simulink model "Id_u_d"  (Simulink 7.1)
settings: Solver=ode4  StartTime=0.0  StopTime=6.0  FixedStep=0.001  RelTol=1e-3
settings Model: Creator=Orlo  LastModifiedBy=Orlo
settings OptimizationCC: InlineInvariantSignals=on
settings DebuggingCC: SaveWithParameterizedLinksMsg=none  SignalResolutionControl=TryResolveAllWithWarning  MultiTaskDSMMsg=warning  MultiTaskCondExecSysMsg=none  StrictBusMsg=None
settings RTWCC: IncludeERTFirstTime=on
settings GRTTargetCC: TargetFcnLib=ansi_tfl_tmw.mat

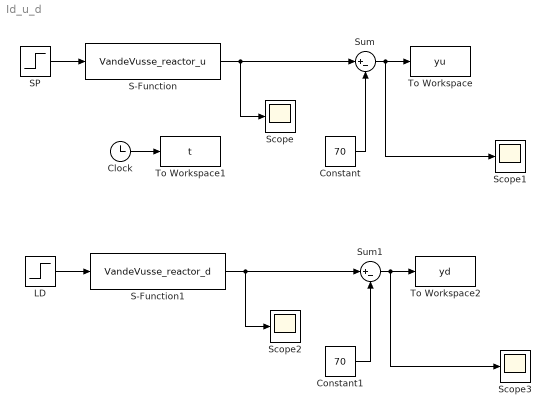
== system Id_u_d ==
  Clock : Clock
      settings: Decimation=10
  Constant : Constant  Value=70  OutDataType=sfix(16)  OutScaling=2^0
  Constant1 : Constant  Value=70  OutDataType=sfix(16)  OutScaling=2^0
  LD : Step  Time=0  After=0  SampleTime=0
  S-Function : S-Function  FunctionName=VandeVusse_reactor_u  Parameters=2.9175, 1.10  EnableBusSupport=off
  S-Function1 : S-Function  FunctionName=VandeVusse_reactor_d  Parameters=2.9175, 1.10  EnableBusSupport=off
  SP : Step  Time=0  After=10  SampleTime=0
  Scope{,1..3} (4 alike) : Scope
      Scope2 settings: SaveName=ScopeData2
      Scope3 settings: SaveName=ScopeData3
  Sum : Sum  Inputs=|+-  OutDataType=sfix(16)  OutScaling=2^0
  Sum1 : Sum  Inputs=|+-  OutDataType=sfix(16)  OutScaling=2^0
  To Workspace : ToWorkspace  VariableName=yu  SampleTime=-1  SaveFormat=Array
  To Workspace1 : ToWorkspace  VariableName=t  SampleTime=-1  SaveFormat=Array
  To Workspace2 : ToWorkspace  VariableName=yd  SampleTime=-1  SaveFormat=Array
  wires:
  SP/1 -> S-Function/1
  S-Function/1 -> Scope/1, Sum/1
  Clock/1 -> To Workspace1/1
  Constant/1 -> Sum/2
  Sum/1 -> To Workspace/1, Scope1/1
  Sum1/1 -> To Workspace2/1, Scope3/1
  Constant1/1 -> Sum1/2
  S-Function1/1 -> Scope2/1, Sum1/1
  LD/1 -> S-Function1/1
